simulink model "transformerparaopen"  (R2020b)
settings: Solver=VariableStepAuto  StartTime=0.0  StopTime=10.0  RelTol=1e-3
libraries: powerlib x12, powerlib_meascontrol x5, eePowerMeasurement x1
settings Model: Creator=admin  LastModifiedBy=admin

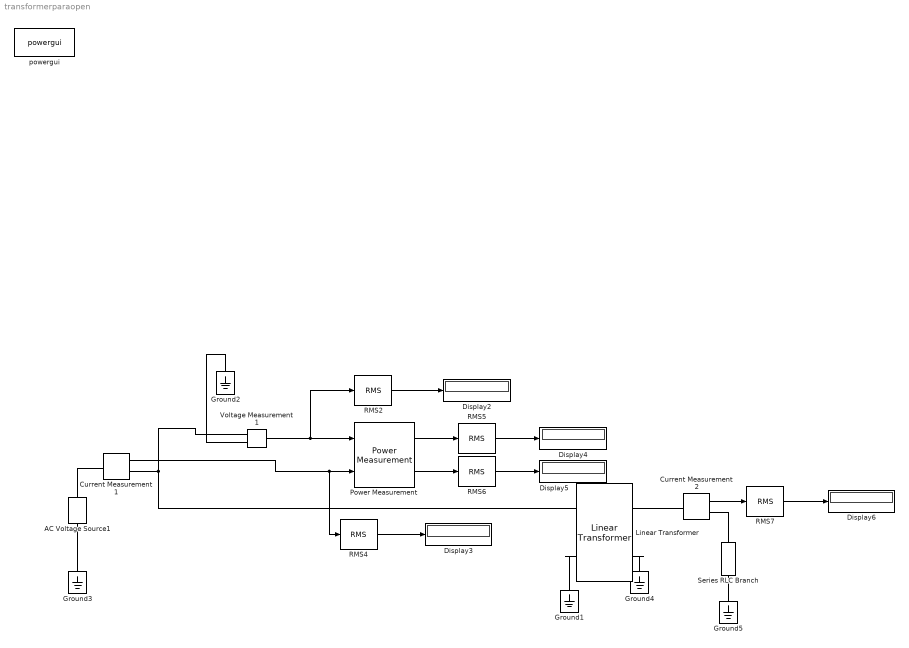
== system transformerparaopen ==
  AC Voltage Source1 : powerlib/Electrical Sources/AC Voltage Source  Amplitude=2400*sqrt(2)  Phase=0  Frequency=50  SampleTime=0  Measurements=Voltage  BusType=swing  Pref=10e3  Qref=0  Qmin=-inf  Qmax=+inf
  Current Measurement1 : powerlib/Measurements/Current Measurement  PhasorSimulation=off  OutputType=Complex  PSBequivalent=0
  Current Measurement2 : powerlib/Measurements/Current Measurement  PhasorSimulation=off  OutputType=Complex  PSBequivalent=0
  Display{2..6} (5 alike) : Display
  Ground{1..5} (5 alike) : powerlib/Elements/Ground  LConnTagsString=a
  Linear Transformer : powerlib/Elements/Linear Transformer  UNITS=SI  NominalPower=[250e6 50 ]  winding1=[220 4.3218 0.45856]  winding2=[110 0.7938 0.084225]  ThreeWindings=off  winding3=[3.15e+05 0.7938 0.084225]  RmLm=[1.0805e+06 2866]  Measurements=None  DataType=on
  Power Measurement : eePowerMeasurement/Power Measurement  LabelModeActiveChoice=Continuous  F=60  K=[0 1 2 3]  Ts=0
      settings: SourceProductBaseCode=PS
  RMS{2,4..7} (5 alike) : powerlib_meascontrol/Measurements/RMS  TrueRMS=on  Freq=50  RMSInit=0  Ts=0
  Series RLC Branch : powerlib/Elements/Series RLC Branch  LConnTagsString=__new0  RConnTagsString=__new0  BranchType=R  Resistance=10000  Inductance=1e-3  SetiL0=off  InitialCurrent=0  Capacitance=1e-6  Setx0=off  InitialVoltage=0  Measurements=None
  Voltage Measurement1 : powerlib/Measurements/Voltage Measurement  PhasorSimulation=off  OutputType=Complex  PSBequivalent=0
  powergui : powerlib/powergui  Priority=1  SimulationMode=Continuous  SampleTime=50e-6  frequency=60  Iterations=50  frequencyindice=50  Pbase=100e6  ErrMax=1e-4  UnitsV=kV  UnitsW=MW  buscounter=0  FunctionMessages=off  echomessages=off  EnableUseOfTLC=off  CurrentSourceSwitches=off  DisableSnubberDevices=off  DisableRonSwitches=off  DisableVfSwitches=off  DisplayEquations=off  AutomaticDiscreteSolvers=off  SolverType=Tustin/Backward Euler (TBE)  Interpol=off  ExternalGateDelay=off  methode=off  Ts=100  x0status=blocks  SPID=on  SwTol=0  HookPort=off  NonlinearTolerance=1e-4  nMaxIteration=100  ContinueOnMaxIteration=off  RestoreLinks=warning  ResistiveCurrentMeasurement=off  Frange=[0:2:500]  Ylog=off  Xlog=on  ShowGrid=off  save=off  variable=ZData  structure=0  ZoomFFT=off  StartTime=0.0  cycles=1  DisplayStyle=1  fundamental=60  FreqAxis=off  MaxFrequency=1000  frequencyindicesteady=1  RmsSteady=1  display=off
  wires:
  Voltage Measurement1/1 -> Power Measurement/1, RMS2/1
  Current Measurement1/1 -> RMS4/1, Power Measurement/2
  RMS4/1 -> Display3/1
  RMS2/1 -> Display2/1
  Power Measurement/1 -> RMS5/1
  Power Measurement/2 -> RMS6/1
  RMS6/1 -> Display5/1
  RMS5/1 -> Display4/1
  RMS7/1 -> Display6/1
  Current Measurement2/1 -> RMS7/1
  connections:
  Current Measurement1/LConn1 -- AC Voltage Source1/RConn1
  Voltage Measurement1/LConn1 -- Linear Transformer/LConn1 -- Current Measurement1/RConn1
  Linear Transformer/LConn2 -- Ground1/LConn1
  Current Measurement2/LConn1 -- Linear Transformer/RConn1
  Ground2/LConn1 -- Voltage Measurement1/LConn2
  Ground3/LConn1 -- AC Voltage Source1/LConn1
  Series RLC Branch/LConn1 -- Current Measurement2/RConn1
  Series RLC Branch/RConn1 -- Ground5/LConn1
  Linear Transformer/RConn2 -- Ground4/LConn1
